simulink model "Analog_Solution"  (R2017a)
settings: Solver=FixedStepDiscrete  StartTime=0.0  StopTime=inf  FixedStep=Ts_main  RelTol=1e-3  EnableMultiTasking=on
InitFcn:
  | clc
  | eval('ContrPrm_v1_1')
model workspace (MAT data in the model file):
  JoyW_sat = 10
values from neighbouring files (symbols this model uses):
  Afilt_Winch = (Amatr_Winch-L_Winch*Cmatr_Winch)    [ContrPrm_v1_1.m]
  AOsat = 10    [ContrPrm_v1_1.m]
  Bfilt_Winch = [L_Winch Bmatr_Winch]    [ContrPrm_v1_1.m]
  Cfilt_Winch = eye(2)    [ContrPrm_v1_1.m]
  Dfilt_Winch = zeros(2)    [ContrPrm_v1_1.m]
  JoyS_gain = 5    [ContrPrm_v1_1.m]
  JoyS_ofst = -2.5    [ContrPrm_v1_1.m]
  JoyS_sat = 9.2    [ContrPrm_v1_1.m]
  JoyW_gain = -5    [ContrPrm_v1_1.m]
  JoyW_ofst = -2.5    [ContrPrm_v1_1.m]
  KspdWinch = 1    [ContrPrm_v1_1.m]
  NPotSpdEst = 3    [ContrPrm_v1_1.m]
  Pot_gain = PotMax/5    (= 0.08)    [ContrPrm_v1_1.m]
  Pot_max = PotMax    (= 0.4)    [ContrPrm_v1_1.m]
  Pot_min = 0    [ContrPrm_v1_1.m]
  Pot_ofst = -0.0558    [ContrPrm_v1_1.m]
  Ts_1ms = 1e-3    (= 0.001)    [ContrPrm_v1_1.m]
  Ts_1s = 1    [ContrPrm_v1_1.m]
  WinchDrumRad = 0.1    [ContrPrm_v1_1.m]
  WinchMotPosAIgain = WinchRevMax/WinchVoltMax*rev2rad    (= 76)    [ContrPrm_v1_1.m]
  WinchMotTorqueMax = 13    [ContrPrm_v1_1.m]
  WinchRefSpdSup = 15/WinchDrumRad    (= 150)    [ContrPrm_v1_1.m]
  WinchTravelMin_m = -2    [ContrPrm_v1_1.m]
  WinchVoltMax = 10    [ContrPrm_v1_1.m]
  x0_Winch = [0;0]    [ContrPrm_v1_1.m]
undefined symbols (not defined in the file or in its folder): datevec, JoyFiltDen, JoyFiltNum, PotPosFiltDen, PotPosFiltNum, WinchPosFiltDen, WinchPosFiltNum, WinchSpdEstFiltDen, WinchSpdEstFiltNum
libraries: slrtlib x10, xpcnilib x6, simulink x6, xpcseriallib x4, xpcwalltimelib x1
(part 3 of 3)

== matlab function Analog_Solution/Inputs/RS232_read/Compass_read/Embedded MATLAB Function ==
  data: in input; GU_Yaw output
function GU_Yaw =Compass_read(in)%#eml

% Message frame: $C357.8P-5.77R1.18T21.8*

% Output: Ground unit Yaw in rad

in_double=double(in);
GU_Yaw=0;

index_end=find(in_double==80);

if ~isempty(index_end)
    ind=index_end(1,1);
    if ind==8;
        GU_Yaw=GU_Yaw+(in_double(7)-48)*1e-1+(in_double(5)-48)+(in_double(4)-48)*1e1+(in_double(3)-48)*1e2;
    elseif ind==7;
        GU_Yaw=GU_Yaw+(in_double(6)-48)*1e-1+(in_double(4)-48)+(in_double(3)-48)*1e1;
    elseif ind==6;
        GU_Yaw=GU_Yaw+(in_double(5)-48)*1e-1+(in_double(3)-48);
    elseif ind==5;
        GU_Yaw=GU_Yaw+(in_double(5)-48)*1e-1;
    end
end

GU_Yaw=GU_Yaw/180*pi;

== matlab function Analog_Solution/Inputs/RS232_read/IMU_read/IMU_data_convert/Subsystem18/Embedded MATLAB Function2 ==
  data: in input; double_out output
function double_out=word2double(in)%#eml

vec1=convert1word(in(1,1));
vec2=convert1word(in(2,1));
vec3=convert1word(in(3,1));
vec4=convert1word(in(4,1));
vec5=convert1word(in(5,1));
vec6=convert1word(in(6,1));
vec7=convert1word(in(7,1));
vec8=convert1word(in(8,1));

temp=[vec1 vec2 vec3 vec4 vec5 vec6 vec7 vec8];

exponent=exp_conv(temp(1,2:12));
signif=signif_conv(temp(1,13:end));
signum=sign_conv(temp(1,1));

if exponent==-1023 
    if signif==0;
        double_out=signum*0;
    else
        double_out=signum*2^-1022*signif;
    end
elseif exponent==1024
    if signif~=0;
        double_out=NaN;
    else
        double_out=signum*Inf;
    end
else
    double_out=signum*2^exponent*(1+signif);
end

function vec=convert1word(in)
vec=zeros(1,8);
ind=uint8(7);

while in>0;
    a=2^ind;
    if in>=a
        vec(1,8-ind)=1;
        in=in-a;
    else
        vec(1,8-ind)=0;
    end
    ind=ind-1;
end

function vec=sign_conv(in)
vec=(-1)^in;

function vec=exp_conv(in)
vec=0;
for ind=1:11;
    vec=vec+in(ind)*2^(11-ind);
end
vec=vec-1023;

function vec=signif_conv(in)
vec=0;
for ind=1:52;
    vec=vec+in(ind)*2^-ind;
end

== matlab function Analog_Solution/Inputs/RS232_read/IMU_read/IMU_data_convert/Subsystem19/Embedded MATLAB Function ==
  data: in input; sing_out output
function sing_out=word2single(in)%#eml

vec1=convert1word(in(1,1));
vec2=convert1word(in(2,1));
vec3=convert1word(in(3,1));
vec4=convert1word(in(4,1));

temp=[vec1 vec2 vec3 vec4];

if sum(temp(1,2:9))==8 && sum(temp(1,10:end))==0;
    sing_out=sign_conv(temp(1,1))*Inf;
elseif sum(temp(1,2:9))==8 && sum(temp(1,10:end))>0;
    sing_out=NaN;
else
    sing_out=sign_conv(temp(1,1))*2^exp_conv(temp(1,2:9))*(1+signif_conv(temp(1,10:end)));
end

function vec=convert1word(in)
vec=zeros(1,8);
ind=uint8(7);

while in>0;
    a=2^ind;
    if in>=a
        vec(1,8-ind)=1;
        in=in-a;
    else
        vec(1,8-ind)=0;
    end
    ind=ind-1;
end

function vec=sign_conv(in)
vec=(-1)^in;

function vec=exp_conv(in)
vec=0;
for ind=1:8;
    vec=vec+in(ind)*2^(8-ind);
end
vec=vec-127;

function vec=signif_conv(in)
vec=0;
for ind=1:23;
    vec=vec+in(ind)*2^-ind;
end

== matlab function Analog_Solution/Inputs/RS232_read/IMU_read/IMU_data_convert/Subsystem19/Embedded MATLAB Function1 ==
  data: in input; sing_out output
function sing_out=word2single(in)%#eml

vec1=convert1word(in(1,1));
vec2=convert1word(in(2,1));
vec3=convert1word(in(3,1));
vec4=convert1word(in(4,1));

temp=[vec1 vec2 vec3 vec4];

if sum(temp(1,2:9))==8 && sum(temp(1,10:end))==0;
    sing_out=sign_conv(temp(1,1))*Inf;
elseif sum(temp(1,2:9))==8 && sum(temp(1,10:end))>0;
    sing_out=NaN;
else
    sing_out=sign_conv(temp(1,1))*2^exp_conv(temp(1,2:9))*(1+signif_conv(temp(1,10:end)));
end

function vec=convert1word(in)
vec=zeros(1,8);
ind=uint8(7);

while in>0;
    a=2^ind;
    if in>=a
        vec(1,8-ind)=1;
        in=in-a;
    else
        vec(1,8-ind)=0;
    end
    ind=ind-1;
end

function vec=sign_conv(in)
vec=(-1)^in;

function vec=exp_conv(in)
vec=0;
for ind=1:8;
    vec=vec+in(ind)*2^(8-ind);
end
vec=vec-127;

function vec=signif_conv(in)
vec=0;
for ind=1:23;
    vec=vec+in(ind)*2^-ind;
end

== matlab function Analog_Solution/Inputs/RS232_read/IMU_read/IMU_data_convert/Subsystem19/Embedded MATLAB Function3 ==
  data: in input; sing_out output
function sing_out=word2single(in)%#eml

vec1=convert1word(in(1,1));
vec2=convert1word(in(2,1));
vec3=convert1word(in(3,1));
vec4=convert1word(in(4,1));

temp=[vec1 vec2 vec3 vec4];

if sum(temp(1,2:9))==8 && sum(temp(1,10:end))==0;
    sing_out=sign_conv(temp(1,1))*Inf;
elseif sum(temp(1,2:9))==8 && sum(temp(1,10:end))>0;
    sing_out=NaN;
else
    sing_out=sign_conv(temp(1,1))*2^exp_conv(temp(1,2:9))*(1+signif_conv(temp(1,10:end)));
end

function vec=convert1word(in)
vec=zeros(1,8);
ind=uint8(7);

while in>0;
    a=2^ind;
    if in>=a
        vec(1,8-ind)=1;
        in=in-a;
    else
        vec(1,8-ind)=0;
    end
    ind=ind-1;
end

function vec=sign_conv(in)
vec=(-1)^in;

function vec=exp_conv(in)
vec=0;
for ind=1:8;
    vec=vec+in(ind)*2^(8-ind);
end
vec=vec-127;

function vec=signif_conv(in)
vec=0;
for ind=1:23;
    vec=vec+in(ind)*2^-ind;
end

== matlab function Analog_Solution/Inputs/RS232_read/IMU_read/IMU_data_convert/Subsystem1/Embedded MATLAB Function2 ==
  data: in input; uint8_out output
function uint8_out=word2uint8(in)%#eml

vec1=convert1word(in(1,1));

temp=[vec1];

uint8_out=uint8_conv(temp);


function vec=uint8_conv(in)
vec=0;
for ind=1:8;
    vec=vec+in(ind)*2^(8-ind);
end

function vec=convert1word(in)
vec=zeros(1,8);
ind=uint8(7);

while in>0;
    a=2^ind;
    if in>=a
        vec(1,8-ind)=1;
        in=in-a;
    else
        vec(1,8-ind)=0;
    end
    ind=ind-1;
end

== matlab function Analog_Solution/Inputs/RS232_read/IMU_read/Data_Check_CRC/Embedded MATLAB Function ==
  data: pBuffer input; CRC_valid output; crc_in input
function CRC_valid  = calcCrc( pBuffer, crc_in )
%CALCCRC pBuffer must be a uint8 array containing the buffer where the CRC
%has to be computed.

bufSize = 143; 
crc_IMU=word2uint16(crc_in);

poly = uint16(hex2dec('8408'));
crc = uint16(0);
for j=1:bufSize
   
    crc = bitxor(crc, uint16(pBuffer(j)));
    for i=1:8
        carry = bitand(crc, 1);
        crc = bitshift(crc,-1);

        if (carry)
            crc = bitxor(crc, poly);
        end
    end
     
end

if (crc == crc_IMU)
    CRC_valid = 1;
else
    CRC_valid = 0;
end


function uint16_out=word2uint16(in)%#eml

vec1=convert1word(in(1,1));
vec2=convert1word(in(2,1));

temp=[vec1 vec2];

uint16_out=uint16_conv(temp);


function vec=uint16_conv(in)
vec=0;
for ind=1:16;
    vec=vec+in(ind)*2^(16-ind);
end

function vec=convert1word(in)
vec=zeros(1,8);
ind=uint8(7);

while in>0;
    a=2^ind;
    if in>=a
        vec(1,8-ind)=1;
        in=in-a;
    else
        vec(1,8-ind)=0;
    end
    ind=ind-1;
end
